simulink model "bldcMotorSimulation"  (R2020b)
settings: Solver=ode23s  StartTime=0.0  StopTime=10.0  MaxStep=1e-2  RelTol=1e-3
InitFcn:
  | bldcParameters
values from neighbouring files (symbols this model uses):
  A = [-R/L, -ki/L ... (first row only)    [bldcParameters.m]
  B = [1/L, 0 ... (first row only)    [bldcParameters.m]
settings Model: Creator=Lindenmaier  LastModifiedBy=Lindenmaier

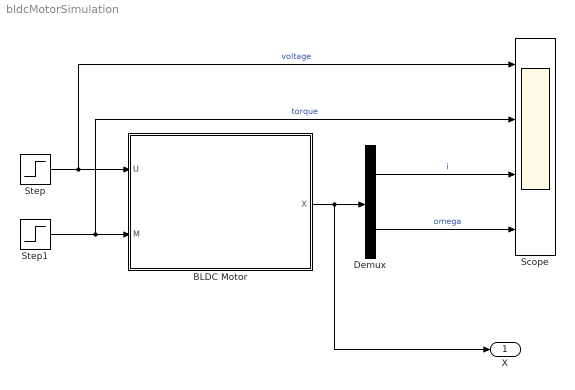
== system bldcMotorSimulation ==
  BLDC Motor : Subsystem
  Demux : Demux  Outputs=2
  Scope : Scope  NumInputPorts=4
  Step : Step  After=5  SampleTime=0
  Step1 : Step  Time=5  After=0.05  SampleTime=0
  X : Outport
  wires:
  Step/1 -> Scope/1, BLDC Motor/1(U)  "voltage"
  Step1/1 -> Scope/2, BLDC Motor/2(M)  "torque"
  BLDC Motor/1(X) -> X/1, Demux/1
  Demux/1 -> Scope/3  "i"
  Demux/2 -> Scope/4  "omega"

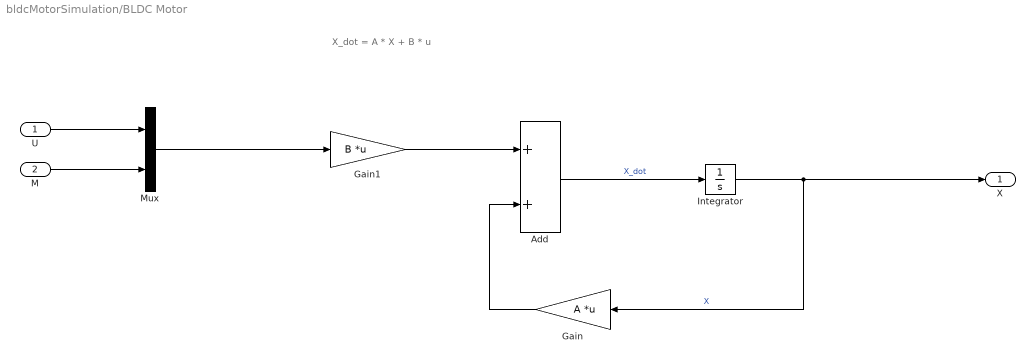
== system bldcMotorSimulation/BLDC Motor ==
  note: X_dot = A * X + B * u
  U : Inport
  M : Inport  Port=2
  Add : Sum
  Gain : Gain  Gain=A  Multiplication=Matrix(K*u)
  Gain1 : Gain  Gain=B  Multiplication=Matrix(K*u)
  Integrator : Integrator  InitialCondition=[0; 0]
  Mux : Mux  Inputs=2
  X : Outport
  wires:
  Integrator/1 -> X/1, Gain/1  "X"
  Add/1 -> Integrator/1  "X_dot"
  Gain/1 -> Add/2
  Gain1/1 -> Add/1
  Mux/1 -> Gain1/1
  U/1 -> Mux/1
  M/1 -> Mux/2
